simulink model "Continuous_Control"  (Simulink 9.1)
settings: Solver=VariableStepAuto  StartTime=0.0  StopTime=20  RelTol=1e-3
settings Model: Creator=syy  LastModifiedBy=syy
settings DataIOCC: SaveFormat=Dataset  ReturnWorkspaceOutputs=on
settings OptimizationCC: LifeSpan=auto
settings DebuggingCC: UnderspecifiedInitializationDetection=Simplified  MergeDetectMultiDrivingBlocksExec=error  SFUnexpectedBacktrackingDiag=error  SFNoUnconditionalDefaultTransitionDiag=error  SFExecutionAtInitializationDiag=warning
settings HardwareCC: ProdBitPerPointer=64  ProdBitPerSizeT=64  ProdBitPerPtrDiffT=64  ProdLargestAtomicFloat=Float  ProdIntDivRoundTo=Zero  ProdEndianess=LittleEndian  ProdWordSize=64  ProdHWDeviceType=Intel->x86-64 (Windows64)
settings ModelReferenceCC: PropagateSignalLabelsOutOfModel=on
settings SFSimCC: SimUseLocalCustomCode=on
settings RTWCC: RTWUseLocalCustomCode=on
settings CodeAppCC: StateflowObjectComments=off
settings GRTTargetCC: TargetLangStandard=C99 (ISO)  CombineOutputUpdateFcns=on  GRTInterface=off
settings ConfigComp: CovMetricSettings=dwe  CovHtmlReporting=off  CovSaveCumulativeToWorkspaceVar=off  CovSaveSingleToWorkspaceVar=off  CovExternalEMLEnable=on

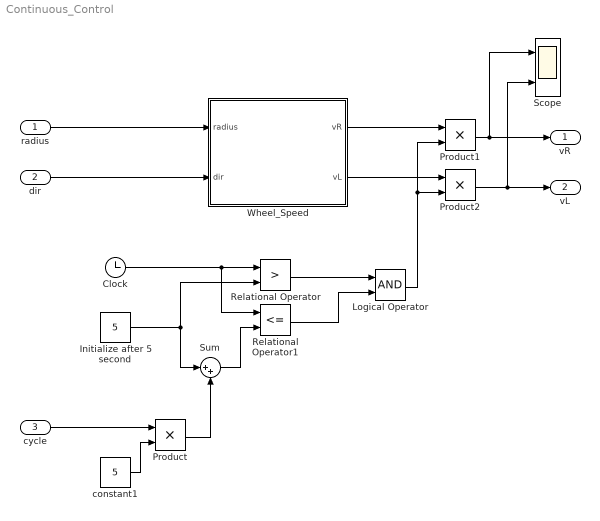
== system Continuous_Control ==
  radius : Inport
  dir : Inport  Port=2
  cycle : Inport  Port=3
  Clock : Clock
  Initialize after 5 second : Constant  Value=5
  Logical Operator : Logic  AllPortsSameDT=off  OutDataTypeStr=boolean
  Product : Product
  Product1 : Product
  Product2 : Product
  Relational Operator : RelationalOperator  Operator=>  OutDataTypeStr=boolean  RndMeth=Simplest
  Relational Operator1 : RelationalOperator  Operator=<=  OutDataTypeStr=boolean  RndMeth=Simplest
  Scope : Scope  NumInputPorts=2
  Sum : Sum  Inputs=|++
  Wheel_Speed : MATLAB Function  TreatAsAtomicUnit=on
  constant1 : Constant  Value=5
  vR : Outport
  vL : Outport  Port=2
  wires:
  radius/1 -> Wheel_Speed/1(radius)
  dir/1 -> Wheel_Speed/2(dir)
  Initialize after 5 second/1 -> Sum/1, Relational Operator/2
  Clock/1 -> Relational Operator1/1, Relational Operator/1
  cycle/1 -> Product/1
  constant1/1 -> Product/2
  Product/1 -> Sum/2
  Sum/1 -> Relational Operator1/2
  Relational Operator/1 -> Logical Operator/1
  Relational Operator1/1 -> Logical Operator/2
  Wheel_Speed/2(vL) -> Product2/1
  Wheel_Speed/1(vR) -> Product1/1
  Product1/1 -> Scope/1, vR/1
  Product2/1 -> Scope/2, vL/1
  Logical Operator/1 -> Product2/2, Product1/2

== matlab function Wheel_Speed ==
  data: radius input double; vR output double; dir input double; vL output double
% 作者：Syy
% 编辑日期：2020/12/29  
function [vR, vL] = Wheel_Speed(radius, dir)
% 该模块直接控制quanser机器人进行圆轨迹的跟踪
% 输入radius为圆的半径，输入dir为圆的方向（0为逆时针，1位顺时针）
 omega = 1.2547;    % 角速度
 d = 0.235;         % 小车直径
 vR = 0; vL = 0;
 if dir == 0
     vR = omega*(radius + d/2);
     vL = omega*(radius - d/2);
 elseif dir == 1
     vR = omega*(radius - d/2);
     vL = omega*(radius + d/2);
 end
